simulink model "tline_sim"  (R2014a)
settings: Solver=ode45  StartTime=0.0  StopTime=10.0  RelTol=1e-3
values from neighbouring files (symbols this model uses):
  tline_sys = sys_class    [create_all_sys.m]
settings Model: Creator=UX31  LastModifiedBy=UX31

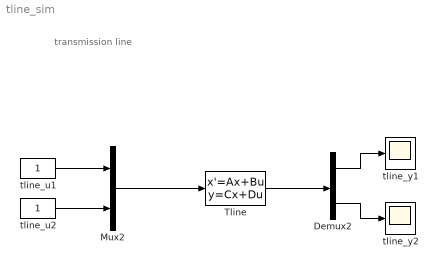
== system tline_sim ==
  note: transmission line
  Demux2 : Demux  Outputs=2
  Mux2 : Mux  Inputs=2
  Tline : StateSpace  A=tline_sys.sys.a  B=tline_sys.sys.b  C=tline_sys.sys.c  D=tline_sys.sys.d  X0=tline_sys.x0_lb
  tline_u1 : Constant
  tline_u2 : Constant
  tline_y1 : Scope
      settings: SaveName=ScopeData5
  tline_y2 : Scope
      settings: SaveName=ScopeData6
  wires:
  Mux2/1 -> Tline/1
  tline_u1/1 -> Mux2/1
  tline_u2/1 -> Mux2/2
  Tline/1 -> Demux2/1
  Demux2/1 -> tline_y1/1
  Demux2/2 -> tline_y2/1
